simulink model "tv"  (R2023b)
settings: Solver=VariableStepAuto  StartTime=0.0  StopTime=10.0  RelTol=1e-3
settings Model: Creator=no  LastModifiedBy=no

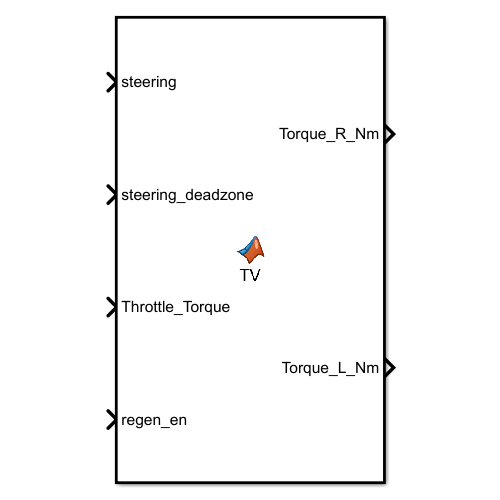
[thumbnail: Simulink's stored preview of the top-level diagram]
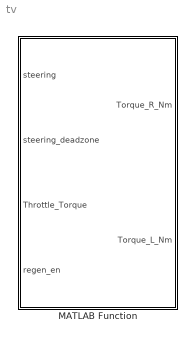
== system tv ==
  MATLAB Function : MATLAB Function  TreatAsAtomicUnit=on

== matlab function tv/MATLAB Function ==
  data: Torque_R_Nm output; Torque_L_Nm output; steering input; steering_deadzone input; Throttle_Torque input; regen_en input
function [Torque_R_Nm, Torque_L_Nm] = TV(steering, steering_deadzone, Throttle_Torque, regen_en)

if abs(steering)<=steering_deadzone %add steering deadzone (º)
    Torque_L_Nm = Throttle_Torque;
    Torque_R_Nm = Throttle_Torque;
    return;
end

d = abs(steering)*0.8-12; %evaluate delta torque for given steering angle
if regen_en
    d=torque;%force torque to be positive to avoid balance issues
end
if s<0 %if steering left, apply full torque to the emotor on the outside
       %and substract the delta from the inside one
    Torque_L_Nm = Throttle_Torque-d;
    Torque_R_Nm = Throttle_Torque;
    return;
end
%opposite case
Torque_L_Nm = Throttle_Torque;
Torque_R_Nm = Throttle_Torque-d;
end
